simulink model "test_VisionModel_v2"  (Simulink 7.6)
settings: Solver=FixedStepDiscrete  StartTime=0.0  StopTime=0  RelTol=1e-3
undefined symbols (not defined in the file or in its folder): black_al, black_au, black_bl, black_bu, blue_al, blue_au, blue_bl, blue_bu, gray, green_al, green_au, green_bl, green_bu, orange_al, orange_au, orange_bl, orange_bu, red_al, red_au, red_bl, red_bu, white_al, white_au, white_bl, white_bu, yellow_al, yellow_au, yellow_bl, yellow_bu
libraries: vipsnks x2, vipsrcs x2
settings Model: Creator=Thing 1  LastModifiedBy=auvt
settings OptimizationCC: InlineParams=on  OptimizeModelRefInitCode=on
settings RTWCC: SystemTargetFile=ert.tlc  GenCodeOnly=on  TemplateMakefile=ert_default_tmf  Description=Real-Time Workshop Embedded Coder  GenerateReport=on  ProcessScript=ert_make_rtw_hook  IncludeHyperlinkInReport=on  LaunchReport=on  TargetLang=C++
settings CodeAppCC: IgnoreCustomStorageClasses=off
settings ERTTargetCC: MultiwordLength=2048  GenerateSampleERTMain=on  IncludeMdlTerminateFcn=off  ERTCustomFileTemplate=example_file_process.tlc  ConvertIfToSwitch=off

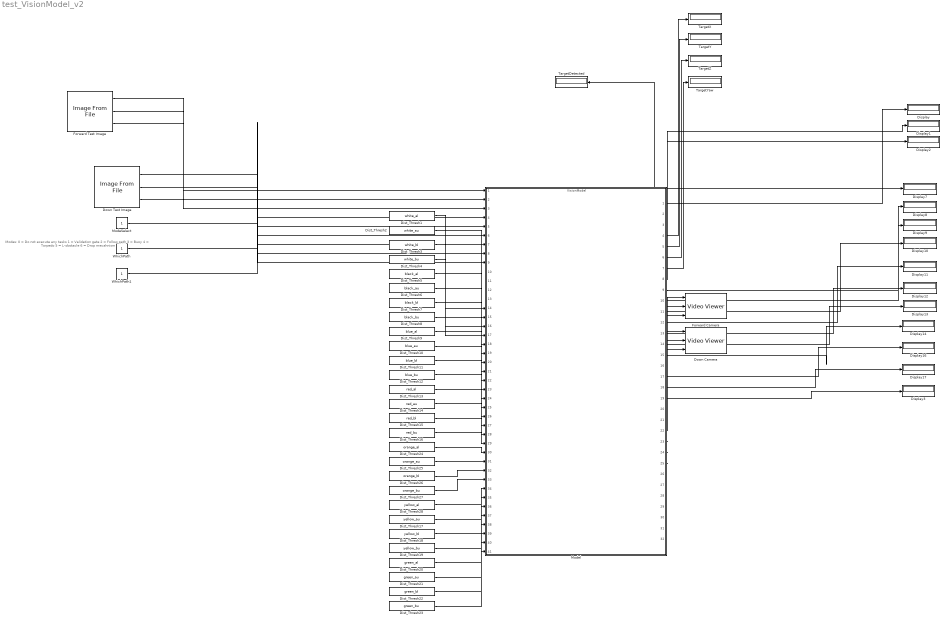
== system test_VisionModel_v2 ==
  note: Modes:
      | 0 = Do not execute any tasks
      | 1 = Validation gate
      | 2 = Follow path
      | 3 = Buoy
      | 4 = Torpedo
      | 5 = L-obstacle
      | 6 = Drop mecahnism
  Display{,1..3,7..14,16..17} (14 alike) : Display
  Dist_Thresh1 : Constant  Value=white_al  SampleTime=-1
  Dist_Thresh10 : Constant  Value=blue_au  SampleTime=-1
  Dist_Thresh11 : Constant  Value=blue_bl  SampleTime=-1
  Dist_Thresh12 : Constant  Value=blue_bu  SampleTime=-1
  Dist_Thresh13 : Constant  Value=red_al  SampleTime=-1
  Dist_Thresh14 : Constant  Value=red_au  SampleTime=-1
  Dist_Thresh15 : Constant  Value=red_bl  SampleTime=-1
  Dist_Thresh16 : Constant  Value=red_bu  SampleTime=-1
  Dist_Thresh17 : Constant  Value=yellow_au  SampleTime=-1
  Dist_Thresh18 : Constant  Value=yellow_bl  SampleTime=-1
  Dist_Thresh19 : Constant  Value=yellow_bu  SampleTime=-1
  Dist_Thresh2 : Constant  Value=white_au  SampleTime=-1
  Dist_Thresh20 : Constant  Value=green_al  SampleTime=-1
  Dist_Thresh21 : Constant  Value=green_au  SampleTime=-1
  Dist_Thresh22 : Constant  Value=green_bl  SampleTime=-1
  Dist_Thresh23 : Constant  Value=green_bu  SampleTime=-1
  Dist_Thresh24 : Constant  Value=orange_al  SampleTime=-1
  Dist_Thresh25 : Constant  Value=orange_au  SampleTime=-1
  Dist_Thresh26 : Constant  Value=orange_bl  SampleTime=-1
  Dist_Thresh27 : Constant  Value=orange_bu  SampleTime=-1
  Dist_Thresh28 : Constant  Value=yellow_al  SampleTime=-1
  Dist_Thresh3 : Constant  Value=white_bl  SampleTime=-1
  Dist_Thresh4 : Constant  Value=white_bu  SampleTime=-1
  Dist_Thresh5 : Constant  Value=black_al  SampleTime=-1
  Dist_Thresh6 : Constant  Value=black_au  SampleTime=-1
  Dist_Thresh7 : Constant  Value=black_bl  SampleTime=-1
  Dist_Thresh8 : Constant  Value=black_bu  SampleTime=-1
  Dist_Thresh9 : Constant  Value=blue_al  SampleTime=-1
  Down Camera : vipsnks/Video Viewer  DialogControllerArgs=DataTag1  inputType=Obsolete7b  imagePorts=Separate color signals  useColorMap=off  colormapValue=gray(256)  specRange=off  minInputVal=0  maxInputVal=255  FigPos=[1011 737 364 553]  AxisZoom=on  trueSizedOnce=off  OpenAtMdlStart=on
  Down Test Image : vipsrcs/Image From File  Tag=vipblks_nd  DialogController=vipDDGCreate  DialogControllerArgs=DataTag2  SystemSampleTime=-1  FileName=/home/auvt/auvc/src/vision/Test_Images/path10.bmp  imagePorts=Separate color signals  Ts=-1  ImageDataType=double  Signed=on  WordLength=16  sdImageDataType=uint(8)  FractionLengthMode=User-defined  FractionLength=15  OutPortLabels=R|G|B
  Forward Camera : vipsnks/Video Viewer  DialogControllerArgs=DataTag4  inputType=Obsolete7b  imagePorts=Separate color signals  useColorMap=off  colormapValue=gray(256)  specRange=off  minInputVal=0  maxInputVal=255  FigPos=[613 732 364 553]  AxisZoom=on  trueSizedOnce=off  OpenAtMdlStart=on
  Forward Test Image : vipsrcs/Image From File  Tag=vipblks_nd  DialogController=vipDDGCreate  DialogControllerArgs=DataTag5  SystemSampleTime=-1  FileName=/home/auvt/auvc/src/vision/Test_Images/L1.PNG  imagePorts=Separate color signals  Ts=-1  ImageDataType=double  Signed=on  WordLength=16  sdImageDataType=uint(8)  FractionLengthMode=User-defined  FractionLength=15  OutPortLabels=R|G|B
  ModeSelect : Constant  SampleTime=-1
  Model : ModelReference  ModelNameDialog=VisionModel  SimulationMode=Accelerator  ModelReferenceVersion=1.504  CopyOfModelName=VisionModel
  TargetDetected : Display
  TargetX : Display
  TargetY : Display
  TargetYaw : Display
  TargetZ : Display
  WhichPath : Constant  SampleTime=-1
  WhichPath1 : Constant  SampleTime=-1
  wires:
  Down Test Image/1 -> Model/4
  Down Test Image/2 -> Model/5
  Down Test Image/3 -> Model/6
  Model/2 -> Display1/1
  Model/8 -> Display7/1
  Model/9 -> Display8/1
  Model/10 -> Display9/1
  Model/11 -> Display10/1
  Model/12 -> Display11/1
  Model/13 -> Display12/1
  Model/14 -> Display13/1
  Model/15 -> Display14/1
  Model/17 -> Display16/1
  Model/18 -> Display17/1
  Forward Test Image/1 -> Model/1
  Forward Test Image/2 -> Model/2
  Forward Test Image/3 -> Model/3
  ModeSelect/1 -> Model/7
  WhichPath/1 -> Model/8
  Model/1 -> Display/1
  Model/3 -> Display2/1
  Model/20 -> Forward Camera/1
  Model/21 -> Forward Camera/2
  Model/22 -> Forward Camera/3
  Model/23 -> Down Camera/1
  Model/24 -> Down Camera/2
  Model/25 -> Down Camera/3
  Model/4 -> TargetX/1
  Model/5 -> TargetY/1
  Model/6 -> TargetZ/1
  Model/7 -> TargetYaw/1
  Model/16 -> TargetDetected/1
  Model/19 -> Display3/1
  WhichPath1/1 -> Model/9
  Dist_Thresh1/1 -> Model/14
  Dist_Thresh2/1 -> Model/15
  Dist_Thresh3/1 -> Model/16
  Dist_Thresh4/1 -> Model/17
  Dist_Thresh5/1 -> Model/18
  Dist_Thresh6/1 -> Model/19
  Dist_Thresh7/1 -> Model/20
  Dist_Thresh8/1 -> Model/21
  Dist_Thresh9/1 -> Model/22
  Dist_Thresh10/1 -> Model/23
  Dist_Thresh11/1 -> Model/24
  Dist_Thresh12/1 -> Model/25
  Dist_Thresh13/1 -> Model/26
  Dist_Thresh14/1 -> Model/27
  Dist_Thresh15/1 -> Model/28
  Dist_Thresh16/1 -> Model/29
  Dist_Thresh24/1 -> Model/30
  Dist_Thresh25/1 -> Model/31
  Dist_Thresh26/1 -> Model/32
  Dist_Thresh27/1 -> Model/33
  Dist_Thresh28/1 -> Model/34
  Dist_Thresh17/1 -> Model/35
  Dist_Thresh18/1 -> Model/36
  Dist_Thresh19/1 -> Model/37
  Dist_Thresh20/1 -> Model/38
  Dist_Thresh21/1 -> Model/39
  Dist_Thresh22/1 -> Model/40
  Dist_Thresh23/1 -> Model/41
